simulink model "lab3_simulink"  (R2018a)
settings: Solver=VariableStepAuto  StartTime=0.0  StopTime=50  RelTol=1e-3
settings Model: Creator=HIBIKI  LastModifiedBy=HIBIKI

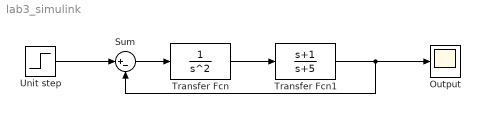
== system lab3_simulink ==
  "Output " : Scope
  Sum : Sum  Inputs=|+-
  Transfer Fcn : TransferFcn  Denominator=[1 0 0]
  Transfer Fcn1 : TransferFcn  Numerator=[1 1]  Denominator=[1 5]
  "Unit step " : Step  SampleTime=0
  wires:
  Transfer Fcn/1 -> Transfer Fcn1/1
  Transfer Fcn1/1 -> Sum/2, "Output "/1
  "Unit step "/1 -> Sum/1
  Sum/1 -> Transfer Fcn/1
